simulink model "HA_sim"  (R2022a)
settings: Solver=ode45  StartTime=0.0  StopTime=Inf  RelTol=1e-3  EnableMultiTasking=on
InitFcn:
  | J = 1.4;
  | l = 1.5;
  | L = 2;
  | m = 5;
  | M = 75;
  | g = 9.81;
libraries: vrlib x5, aerolibanimutils x1
Description:
  | Simulink(R) 3D Animation(TM) - Tutorial #3
  | 
  | Tutorial model to be used for 3D World Editor authoring example in the documentation.
  | After creating the virtual world according to the instructions in the documentation, include the VR block
  | in the model and connect B1, B2 coordinates and S scaling to corresponding nodes in
  | the virtual world.
settings Model: ExtModeTrigMode=oneshot  ExtModeArmWhenConnect=off  Creator=The MathWorks, Inc.  LastModifiedBy=vcichella
settings SolverCC: AlgebraicLoopSolver=TrustRegion
settings DataIOCC: LimitDataPoints=on  SaveFormat=Array  SaveOutput=off  SaveTime=off  ReturnWorkspaceOutputs=off  SignalLoggingName=logsOut
settings OptimizationCC: BooleanDataType=off  ExpressionDepthLimit=2147483647  InitFltsAndDblsToZero=on  LifeSpan=inf
settings DebuggingCC: UnderspecifiedInitializationDetection=Classic  MergeDetectMultiDrivingBlocksExec=none  CheckExecutionContextPreStartOutputMsg=on  SignalResolutionControl=TryResolveAllWithWarning  MultiTaskDSMMsg=warning  MultiTaskCondExecSysMsg=none  FcnCallInpInsideContextMsg=warning  UnconnectedInputMsg=warning  UnconnectedOutputMsg=warning  UnconnectedLineMsg=warning  StateNameClashWarn=warning  SymbolicDimsDataTypeCodeGenerationDiagnostic=none  SFUnexpectedBacktrackingDiag=warning  SFNoUnconditionalDefaultTransitionDiag=warning  SFExecutionAtInitializationDiag=none  SFMachineParentedDataDiag=warning  ArithmeticOperatorsInVariantConditions=warning
settings HardwareCC: ProdBitPerPointer=32  ProdBitPerSizeT=32  ProdBitPerPtrDiffT=32  ProdLargestAtomicFloat=None  ProdIntDivRoundTo=Undefined  ProdEndianess=Unspecified  ProdWordSize=32  ProdHWDeviceType=32-bit Generic  TargetUnknown=on
settings ModelReferenceCC: UpdateModelReferenceTargets=IfOutOfDate  PropagateSignalLabelsOutOfModel=off
settings SFSimCC: SimUseLocalCustomCode=off  CustomCodeUndefinedFunction=UseInterfaceOnly
settings RTWCC: RTWUseLocalCustomCode=off
settings CodeAppCC: StateflowObjectComments=on
settings GRTTargetCC: TargetFcnLib=ansi_tfl_tmw.mat  TargetLangStandard=C89/C90 (ANSI)  CombineOutputUpdateFcns=off  GRTInterface=on
settings ConfigComp: CovMetricSettings=d  CovSaveCumulativeToWorkspaceVar=on  CovSaveSingleToWorkspaceVar=on  CovExternalEMLEnable=off  CovSFcnEnable=off

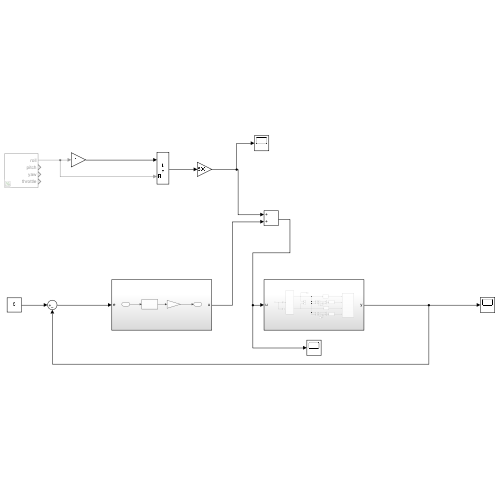
[thumbnail: Simulink's stored preview of the top-level diagram]
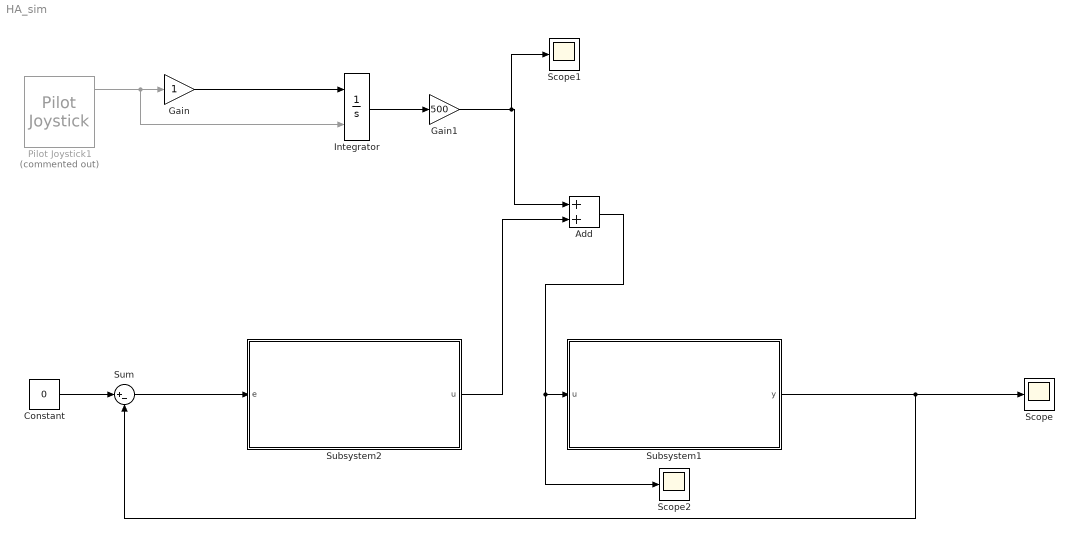
== system HA_sim ==
  Add : Sum
  Constant : Constant  Value=0
  Gain : Gain
  Gain1 : Gain  Gain=500
  Integrator : Integrator  ExternalReset=either
  Pilot Joystick1 : aerolibanimutils/Pilot Joystick  Commented=on  JoystickID=Joystick1  OutputConfiguration=FourAxis  SampleTime=1/30
  Scope : Scope
  Scope1 : Scope
  Scope2 : Scope
  Subsystem1 : Subsystem
  Subsystem2 : Subsystem
  Sum : Sum  Inputs=|+-
  wires:
  Pilot Joystick1/1 -> Integrator/2, Gain/1
  Sum/1 -> Subsystem2/1(e)
  Constant/1 -> Sum/1
  Subsystem1/1(y) -> Scope/1, Sum/2
  Gain/1 -> Integrator/1
  Integrator/1 -> Gain1/1
  Gain1/1 -> Scope1/1, Add/1
  Add/1 -> Scope2/1, Subsystem1/1(u)
  Subsystem2/1(u) -> Add/2

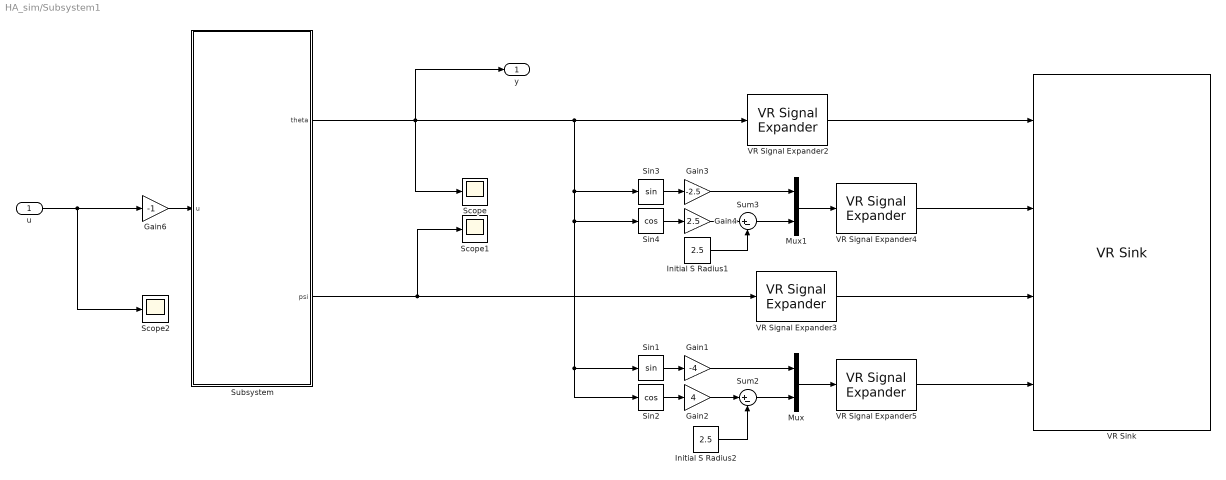
== system HA_sim/Subsystem1 ==
  u : Inport
  Gain1 : Gain  Gain=-4
  Gain2 : Gain  Gain=4
  Gain3 : Gain  Gain=-2.5
  Gain4 : Gain  Gain=2.5
  Gain6 : Gain  Gain=-1
  Initial S Radius1 : Constant  Value=2.5
  Initial S Radius2 : Constant  Value=2.5
  Mux : Mux  Inputs=2
  Mux1 : Mux  Inputs=2
  Scope : Scope
  Scope1 : Scope
  Scope2 : Scope
  Sin1 : Trigonometry
  Sin2 : Trigonometry  Operator=cos
  Sin3 : Trigonometry
  Sin4 : Trigonometry  Operator=cos
  Subsystem : Subsystem
  Sum2 : Sum  Inputs=|+-  InputSameDT=on  SaturateOnIntegerOverflow=on  OutDataTypeStr=Inherit: Same as first input
  Sum3 : Sum  Inputs=|+-  InputSameDT=on  SaturateOnIntegerOverflow=on  OutDataTypeStr=Inherit: Same as first input
  VR Signal Expander2 : vrlib/VR Signal Expander  outwidth=4  outidx=4
  VR Signal Expander3 : vrlib/VR Signal Expander  outwidth=4  outidx=4
  VR Signal Expander4 : vrlib/VR Signal Expander  outwidth=3  outidx=[1 2]
  VR Signal Expander5 : vrlib/VR Signal Expander  outwidth=3  outidx=[1 2]
  VR Sink : vrlib/VR Sink  InstantiateOnLoad=on  SampleTime=0.1  ViewEnable=on  RemoteChange=off  RemoteView=off  FieldsWritten=B1.rotation.4.1.1.double#B1.translation.3.1.1.double#B2.rotation.4.1.1.double#B2.translation.3.1.1.double  WorldFileName=vr_highwire.x3d  WorldDescription=vr_highwire  AutoView=on  VideoDimensions=[]  AllowVariableSize=off  FigureProperties="{'Position', 'Name', 'Viewpoint', 'CameraBound', 'CameraDirection', 'CameraPosition', 'CameraUpVector', 'ZoomFactor', 'Antialiasing', 'Headlight', 'Lighting', 'NavPanel', 'Sound', 'StatusBar', 'Stereo3D', 'Stereo3DCameraOffset', 'Stereo3DHIT', 'ToolBar', 'Textures', 'Transparency', 'Triad', 'Wireframe', 'NavZones', 'NavMode', 'NavSpeed', 'CaptureFileFormat', 'CaptureFileName', 'Record2DCompressMethod', 'Record2DCompressQuality', 'Record2D', 'Record2DFileName', 'Record2DFPS'; [2.0000000000000000e+00   9.2000000000000000e+01   5.7600000000000000e+02   3.5000000000000000e+02], 'vr_highwire', '', 'on', [0.0000000000000000e+00   0.0000000000000000e+00  -1.0000000000000000e+00], [0.0000000000000000e+00  -6.5784311294555664e-01   1.3048258590698241e+01], [0.0000000000000000e+00   1.0000000000000000e+00   0.0000000000000000e+00], [1.0000000000000000e+00], 'on', 'on', 'on', 'halfbar', 'on', 'on', 'off', [1.0000000149011612e-01], [0.0000000000000000e+00], 'on', 'on', 'on', 'none', 'off', 'off', 'fly', 'normal', 'tif', '%f_anim_%n.tif', 'auto', [7.5000000000000000e+01], 'off', '%f_anim_%n.avi', 'auto'}"
  y : Outport
  wires:
  VR Signal Expander5/1 -> VR Sink/4
  Initial S Radius2/1 -> Sum2/2
  Subsystem/2(psi) -> Scope1/1, VR Signal Expander3/1
  Sin2/1 -> Gain2/1
  Gain6/1 -> Subsystem/1(u)
  Gain2/1 -> Sum2/1
  Subsystem/1(theta) -> y/1, Scope/1, Sin3/1, Sin4/1, Sin2/1, Sin1/1, VR Signal Expander2/1
  Mux/1 -> VR Signal Expander5/1
  Gain1/1 -> Mux/1
  Sin4/1 -> Gain4/1
  Sin3/1 -> Gain3/1
  Sum2/1 -> Mux/2
  Mux1/1 -> VR Signal Expander4/1
  Initial S Radius1/1 -> Sum3/2
  VR Signal Expander2/1 -> VR Sink/1
  Sin1/1 -> Gain1/1
  Gain4/1 -> Sum3/1
  Sum3/1 -> Mux1/2
  u/1 -> Scope2/1, Gain6/1
  Gain3/1 -> Mux1/1
  VR Signal Expander4/1 -> VR Sink/2
  VR Signal Expander3/1 -> VR Sink/3

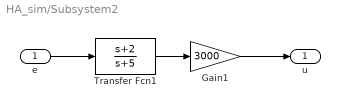
== system HA_sim/Subsystem2 ==
  e : Inport
  Gain1 : Gain  Gain=3000
  Transfer Fcn1 : TransferFcn  Numerator=[1 2]  Denominator=[1 5]
  u : Outport
  wires:
  e/1 -> Transfer Fcn1/1
  Transfer Fcn1/1 -> Gain1/1
  Gain1/1 -> u/1

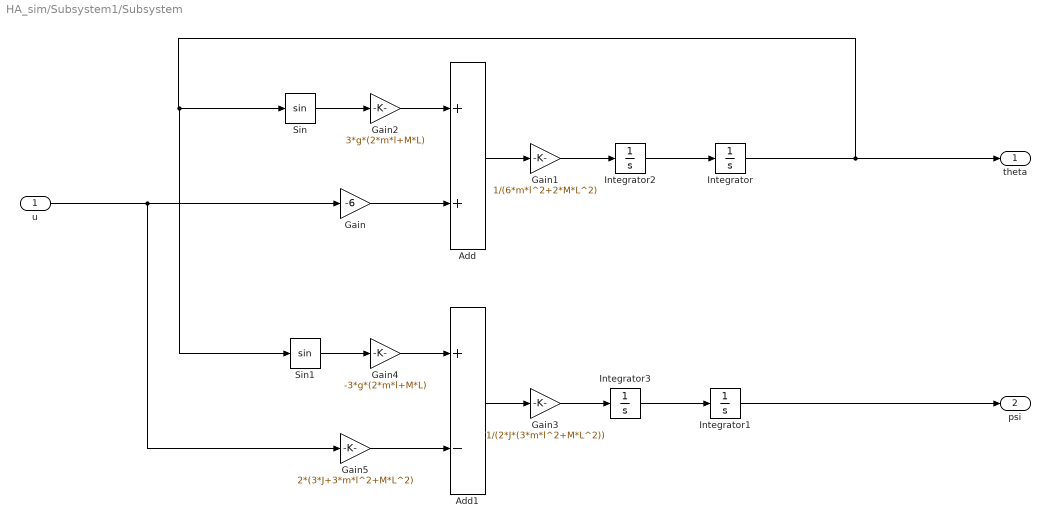
== system HA_sim/Subsystem1/Subsystem ==
  u : Inport
  Add : Sum
  Add1 : Sum  Inputs=+-
  Gain : Gain  Gain=-6
  Gain1 : Gain  Gain=1/(6*m*l^2+2*M*L^2)
  Gain2 : Gain  Gain=3*g*(2*m*l+M*L)
  Gain3 : Gain  Gain=1/(2*J*(3*m*l^2+M*L^2))
  Gain4 : Gain  Gain=-3*g*(2*m*l+M*L)
  Gain5 : Gain  Gain=2*(3*J+3*m*l^2+M*L^2)
  Integrator : Integrator  InitialCondition=pi/1000
  Integrator1 : Integrator
  Integrator2 : Integrator
  Integrator3 : Integrator
  Sin : Trigonometry
  Sin1 : Trigonometry
  theta : Outport
  psi : Outport  Port=2
  wires:
  Integrator3/1 -> Integrator1/1
  Integrator1/1 -> psi/1
  Integrator2/1 -> Integrator/1
  Integrator/1 -> Sin1/1, Sin/1, theta/1
  Add/1 -> Gain1/1
  u/1 -> Gain5/1, Gain/1
  Gain/1 -> Add/2
  Gain1/1 -> Integrator2/1
  Sin/1 -> Gain2/1
  Gain2/1 -> Add/1
  Add1/1 -> Gain3/1
  Gain3/1 -> Integrator3/1
  Sin1/1 -> Gain4/1
  Gain4/1 -> Add1/1
  Gain5/1 -> Add1/2
